simulink model "center_seeking_process"  (Simulink 3.00)
libraries: mathlib x1, modellib x1

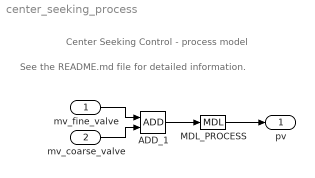
== system center_seeking_process ==
  note: See the README.md file for detailed information.
  note: Center Seeking Control - process model
  mv_fine_valve : Inport  Port=1
  mv_coarse_valve : Inport  Port=2
  ADD_1 : mathlib/ADD
  MDL_PROCESS : modellib/MDL  k0=10  del=0  tau1=3  tau2=5  nmax=100
  pv : Outport  Port=1
  wires:
  ADD_1/1 -> MDL_PROCESS/1
  MDL_PROCESS/1 -> pv/1
  mv_coarse_valve/1 -> ADD_1/2
  mv_fine_valve/1 -> ADD_1/1
